simulink model "HydraulicLinearMotorArm(conflicted copy 04-22-2025 09_51_49)"  (R2024a)
settings: Solver=VariableStepAuto  StartTime=0.0  StopTime=inf  MaxStep=0.033333333333333333  RelTol=1e-3
libraries: arduinolib x10, arduinosensorlib x2, aerolibanimutils x1
settings Model: Creator=Akbar  LastModifiedBy=Akbar

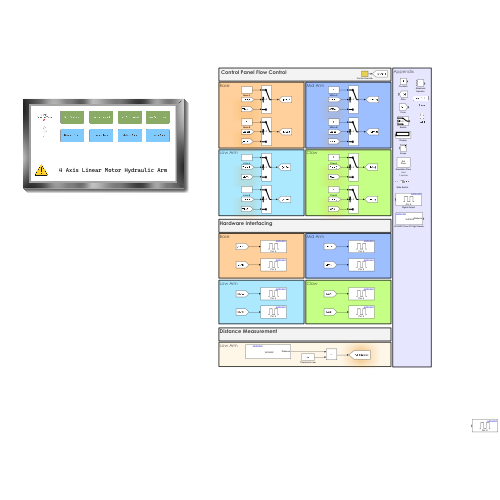
[thumbnail: Simulink's stored preview of the top-level diagram]
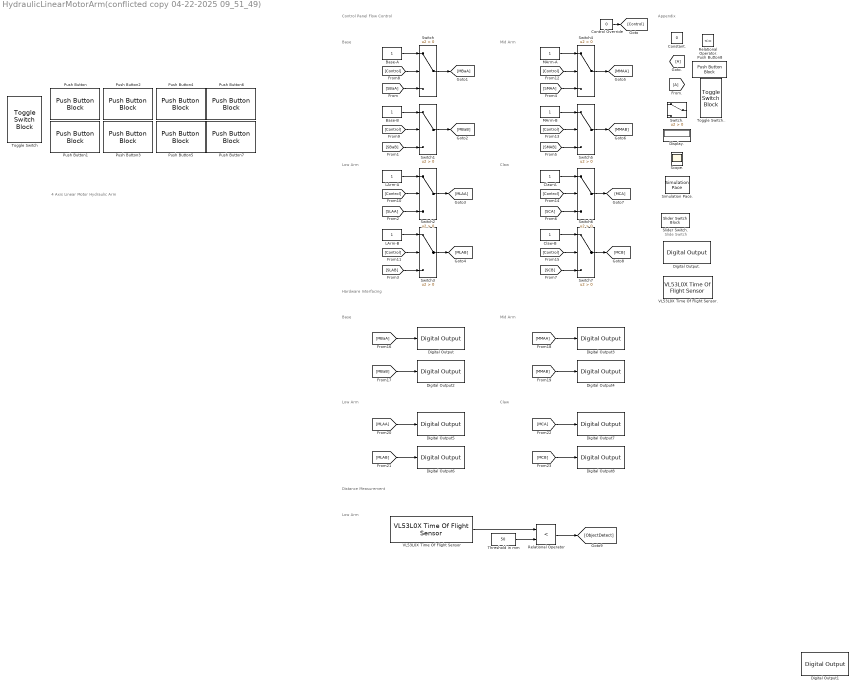
== system HydraulicLinearMotorArm(conflicted copy 04-22-2025 09_51_49) ==
  note: 4 Axis Linear Motor Hydraulic Arm
  note: Slide Switch
  note: Appendix
  note: Control Panel Flow Control
  note: Base
  note: Low Arm
  note: Mid Arm
  note: Claw
  note: Claw
  note: Hardware Interfacing
  note: Low Arm
  note: Mid Arm
  note: Base
  note: Distance Measurement
  note: Low Arm
  Base-A : Constant
  Base-B : Constant
  Claw-A : Constant
  Claw-B : Constant
  Constant. : Constant  Value=0
  Control Override : Constant  Value=0
  Digital Output{,1..8} (9 alike) : arduinolib/Digital Output  pinNumber=9  Direction=output  blockPlatform=arduino
  Digital Output. : arduinolib/Digital Output  pinNumber=9  Direction=output  blockPlatform=arduino
  Display. : Display
  From. : From
  Goto. : Goto
  LArm-A : Constant
  LArm-B : Constant
  MArm-A : Constant
  MArm-B : Constant
  Push Button : PushButtonBlock  ButtonText=Base Clockwise  OffValue=1.000000
  Push Button1 : PushButtonBlock  ButtonText=Base AntiClock  OffValue=1.000000
  Push Button2 : PushButtonBlock  ButtonText=Low Arm Forward  OffValue=1.000000
  Push Button3 : PushButtonBlock  ButtonText=Low Arm Back  OffValue=1.000000
  Push Button4 : PushButtonBlock  ButtonText=Mid Arm Forward  OffValue=1.000000
  Push Button5 : PushButtonBlock  ButtonText=Mid Arm Back  OffValue=1.000000
  Push Button6 : PushButtonBlock  ButtonText=Low Arm Forward  OffValue=1.000000
  Push Button7 : PushButtonBlock  ButtonText=Low Arm Back  OffValue=1.000000
  Push Button8 : PushButtonBlock  ButtonText=Push Button
  Relational Operator : RelationalOperator  Operator=<  OutDataTypeStr=boolean  RndMeth=Simplest  InputSameDT=off
  Relational Operator. : RelationalOperator  Operator=<=  OutDataTypeStr=boolean  RndMeth=Simplest  InputSameDT=off
  Scope. : Scope
  Simulation Pace. : aerolibanimutils/Simulation Pace  SimulationPace=1  SleepMode=Auto  OutputPaceError=off  SampleTime=1/30
  Slider Switch. : SliderSwitchBlock  LabelPosition=Hide
      settings: Values={{'Off', 'On'}, [0 1]}
  Switch{,1..7} (8 alike) : Switch  Criteria=u2 > Threshold  SaturateOnIntegerOverflow=off  InputSameDT=off
  Switch. : Switch  Criteria=u2 > Threshold  SaturateOnIntegerOverflow=off  InputSameDT=off
  Threshold in mm : Constant  Value=50
  Toggle Switch : ToggleSwitchBlock
      settings: Values={{'Off', 'On'}, [0 1]}
  Toggle Switch.. : ToggleSwitchBlock  LabelPosition=Hide
      settings: Values={{'Switch', 'Toggle'}, [0 1]}
  VL53L0X Time Of Flight Sensor : arduinosensorlib/VL53L0X Time Of Flight Sensor  I2CModule=0  I2CAddress=0x29  BitRate=1000000  RangingMode=Default  SampleTime=-1
  VL53L0X Time Of Flight Sensor. : arduinosensorlib/VL53L0X Time Of Flight Sensor  I2CModule=0  I2CAddress=0x29  BitRate=1000000  RangingMode=Default  SampleTime=-1
  wires:
  Base-A/1 -> Switch/1
  Base-B/1 -> Switch1/1
  LArm-A/1 -> Switch2/1
  LArm-B/1 -> Switch3/1
  [SBaA] -> Switch/3
  [SBaB] -> Switch1/3
  [SLAA] -> Switch2/3
  [SLAB] -> Switch3/3
  MArm-B/1 -> Switch5/1
  MArm-A/1 -> Switch4/1
  [SMAA] -> Switch4/3
  [SMAB] -> Switch5/3
  Claw-B/1 -> Switch7/1
  [SCA] -> Switch6/3
  [SCB] -> Switch7/3
  Claw-A/1 -> Switch6/1
  Control Override/1 -> [Control]
  [Control] -> Switch/2
  [Control] -> Switch1/2
  [Control] -> Switch2/2
  [Control] -> Switch3/2
  [Control] -> Switch4/2
  [Control] -> Switch5/2
  [Control] -> Switch6/2
  [Control] -> Switch7/2
  Switch/1 -> [MBaA]
  Switch1/1 -> [MBaB]
  Switch2/1 -> [MLAA]
  Switch3/1 -> [MLAB]
  Switch4/1 -> [MMAA]
  Switch5/1 -> [MMAB]
  Switch6/1 -> [MCA]
  Switch7/1 -> [MCB]
  [MBaB] -> Digital Output2/1
  [MBaA] -> Digital Output/1
  [MMAA] -> Digital Output3/1
  [MMAB] -> Digital Output4/1
  [MLAA] -> Digital Output5/1
  [MLAB] -> Digital Output6/1
  [MCA] -> Digital Output7/1
  [MCB] -> Digital Output8/1
  VL53L0X Time Of Flight Sensor/1 -> Relational Operator/1
  Threshold in mm/1 -> Relational Operator/2
  Relational Operator/1 -> [ObjectDetect]
